simulink model "GRM_HIL_Simple"  (R2019b)
settings: Solver=ode5  StartTime=0.0  StopTime=10.0  FixedStep=0.001  RelTol=1e-3
values from neighbouring files (symbols this model uses):
  HIL_Sample_Time = 0.001    [initialize_GRM_HIL.m]
undefined symbols (not defined in the file or in its folder): Serial_Port, Standard_Devices
libraries: lib_Serial_PIX x2, sldrtlib x1
settings Model: Creator=guy-m  LastModifiedBy=guy-m
settings RTWCC: Description=Simulink Desktop Real-Time  SystemTargetFile=sldrt.tlc  TemplateMakefile=sldrt.tmf  RTWCompilerOptimization=on
settings CodeAppCC: MaxIdLength=95
settings SimulinkDesktopRealTimeCC: TargetPreCompLibLocation=C:\Program Files\MATLAB\R2019b\toolbox\sldrt\lib\win64  PreserveStateflowLocalDataDimensions=off

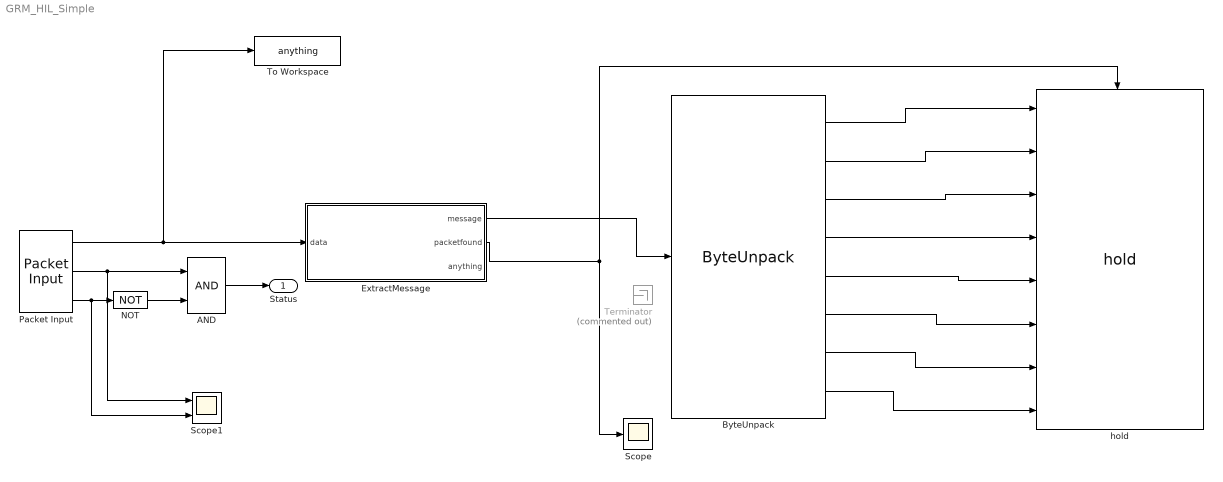
== system GRM_HIL_Simple ==
  AND : Logic  IconShape=distinctive  AllPortsSameDT=off  OutDataTypeStr=boolean
  ByteUnpack : lib_Serial_PIX/Serial_Recieve_from_Pixhawk/input_hold/ByteUnpack  SystemSampleTime=-1  Latency=0  AutoFrameSizeCalculation=off
  ExtractMessage : MATLAB Function  AncestorBlock=lib_Serial_PIX/Serial_Recieve_from_Pixhawk/input_hold/ExtractMessage  TreatAsAtomicUnit=on
  NOT : Logic  Operator=NOT  IconShape=distinctive  AllPortsSameDT=off  OutDataTypeStr=boolean
  Packet Input : sldrtlib/Packet Input  SampleTime=HIL_Sample_Time  MaxMissedTicks=100  ShowMissedTicks=off  YieldWhenWaiting=on  DrvName=Standard_Devices/Serial_Port  DrvAddress=11  DrvOptions=[115200 8 0 0 0 0 0 1]  PacketSize=78  DataTypes='78*uint8'  ShowReady=on  ShowError=on  PacketID=1  ByteOrder=1  ShowTimestamp=off
      settings: AttributesFormatString=Serial Port [11]  SourceProductName=Simulink Desktop Real-Time
  Scope : Scope
  Scope1 : Scope  NumInputPorts=2
  Terminator : Terminator  Commented=on
  To Workspace : ToWorkspace  VariableName=anything  SaveFormat=Timeseries  SampleTime=-1
  hold : lib_Serial_PIX/Serial_Recieve_from_Pixhawk/input_hold/hold  SystemSampleTime=-1  Latency=0  AutoFrameSizeCalculation=off
  Status : Outport  VectorParamsAs1DForOutWhenUnconnected=off
  wires:
  Packet Input/3 -> Scope1/2, NOT/1
  Packet Input/2 -> Scope1/1, AND/1
  AND/1 -> Status/1
  NOT/1 -> AND/2
  ExtractMessage/1(message) -> ByteUnpack/1
  Packet Input/1 -> To Workspace/1, ExtractMessage/1(data)
  ByteUnpack/3 -> hold/3
  ByteUnpack/4 -> hold/4
  ExtractMessage/2(packetfound) -> Scope/1, hold/Enable
  ByteUnpack/6 -> hold/6
  ByteUnpack/1 -> hold/1
  ByteUnpack/2 -> hold/2
  ByteUnpack/8 -> hold/8
  ByteUnpack/7 -> hold/7
  ByteUnpack/5 -> hold/5

== matlab function GRM_HIL_Simple/ExtractMessage ==
  data: data input uint8 size=[78 1]; message output uint8 size=[1 64]; packetfound output; anything output
function [message,packetfound,anything] = ExtractMessage(data)
    
    %specify size and type of input and output data in data manager!!
    
    data = data';
    anything = false;
    expected_message_length = 64; % specify!!
    expected_header = [5 5];      % specify!!
    expected_header_length = length(expected_header);
    expected_packet_length = expected_message_length + expected_header_length;
    
    packet = uint8(zeros(1,expected_message_length));
    packetfound = false;
    
    %% locate packet in data
    
    % First, find possible header start locations; i.e., match the first element in the
    % header.
    start = find(data==expected_header(1));
    
    % Next remove start values that are too close to the end to possibly match
    % the header.
    endVals = start+expected_header_length-1;
    start(endVals>length(data)) = [];
    
    % Next, loop over elements of header, usually much shorter than length of
    % array, to check which possible header start locations are valid still.
    for pattval = 2:expected_header_length
        % check viable locations in array
        locs = expected_header(pattval) == data(start+pattval-1);
        % delete false ones from indices
        start(~locs) = [];
    end
    
    %Packet = Data - Header
    if ~isempty(start)
        for i = 1:(length(start)-1)
            %Verify if the size of data between 2 consecutive header start
            %indices is equal to the expectedPacketSize
            if isequal(start(i+1)-start(i),expected_packet_length)
            
                %Extract the packet by stripping the header from the data
                packet = data(start(i)+expected_header_length:start(i+1)-1);
                if ~isequal(length(packet),(expected_packet_length-expected_header_length))
                    error('ERROR:Wrong packet size');
                end
            
                %Once a valid packet is found, exit the for loop
                packetfound = true;
                break;
            else
                continue
            end
        end
    else
        packetfound = false;
    end
    
    
    
    %% extract message
    
    message = uint8(packet);
    
    
    
    
    
    
end
